simulink library "ControLibrary"  (R2015b)
settings: Solver=ode45  SolverMode=SingleTasking  StartTime=0.0  StopTime=10.0  RelTol=1e-3
values from neighbouring files (symbols this model uses):
  ControlSampleTime = 1/8000    (= 0.000125)    [initTPHardware.m]
  DCCC = initDCCC(LCL,SM)    [Sim_TP3_VSM_init.m]    (also in initDCCC.m = initHSS(LCL,SM))
undefined symbols (not defined in the file or in its folder): CCCTRL, DiscIntNeverNeededParam, VSMCTRL
undefined symbols (not defined in the file): HSS, VSMCC
libraries: FriedrichLibrary x46, simulink x23, simulink_extras x4, ControLibrary x2, ctrl_basic x2
(part 2 of 4)

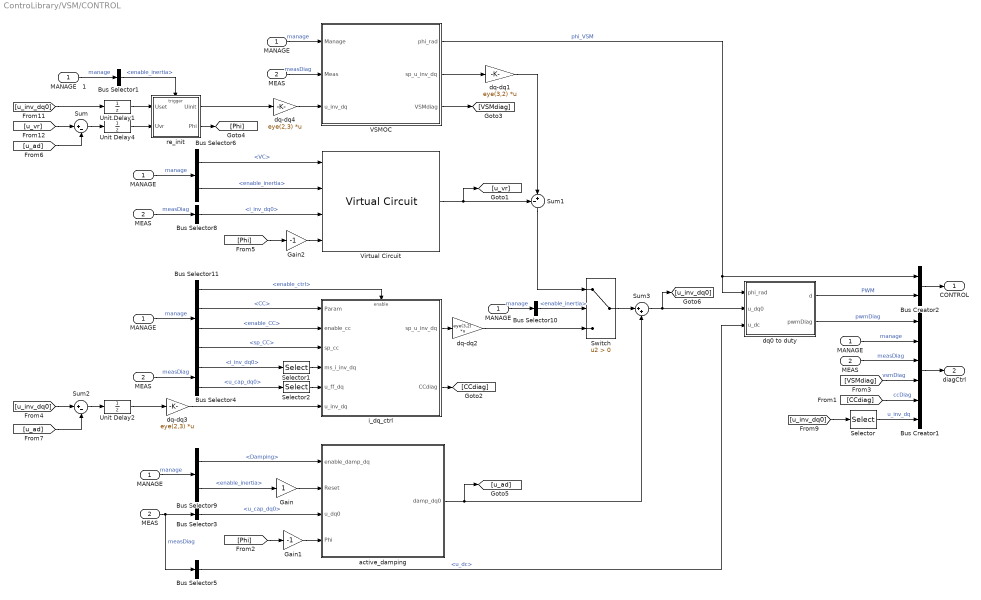
== system ControLibrary/VSM/CONTROL ==
  MANAGE : Inport
  MEAS : Inport  Port=2
  "  MANAGE " : InportShadow
  "  MEAS " : InportShadow  Port=2
  "  MEAS  " : InportShadow  Port=2
  " MANAGE" : InportShadow
  " MEAS" : InportShadow  Port=2
  Bus Creator1 : BusCreator  Inputs=6
  Bus Creator2 : BusCreator  Inputs=2
  Bus Selector1 : BusSelector  OutputSignals=enable_VSM.enable_inertia
  Bus Selector10 : BusSelector  OutputSignals=enable_VSM.enable_inertia
  Bus Selector11 : BusSelector  OutputSignals=enable_VSM.enable_ctrl,Param.CC,enable_CC,sp_CC
  Bus Selector3 : BusSelector  OutputSignals=u_cap.u_cap_dq0
  Bus Selector4 : BusSelector  OutputSignals=i_inv.i_inv_dq0,u_cap.u_cap_dq0
  Bus Selector5 : BusSelector  OutputSignals=u_dc
  Bus Selector6 : BusSelector  OutputSignals=Param.VC,enable_VSM.enable_inertia
  Bus Selector8 : BusSelector  OutputSignals=i_inv.i_inv_dq0
  Bus Selector9 : BusSelector  OutputSignals=Param.Damping,enable_VSM.enable_inertia
  Gain : Gain
  Gain1 : Gain  Gain=-1
  Gain2 : Gain  Gain=-1
  "MANAGE  " : InportShadow
  "MANAGE   " : InportShadow
  "MANAGE    " : InportShadow
  MANAGE   1 : InportShadow
  "MEAS " : InportShadow  Port=2
  Selector : Selector  InputPortWidth=3  IndexOptions=Index vector (dialog)  Indices=[1 2]  OutputSizes=1
  Selector1 : Selector  InputPortWidth=3  IndexOptions=Index vector (dialog)  Indices=[1 2]  OutputSizes=1
  Selector2 : Selector  InputPortWidth=3  IndexOptions=Index vector (dialog)  Indices=[1 2]  OutputSizes=1
  Sum : Sum  Inputs=|+-
  Sum1 : Sum  Inputs=-+|
  Sum2 : Sum  Inputs=|+-
  Sum3 : Sum  Inputs=|++
  Switch : Switch  Criteria=u2 > Threshold
  Unit Delay1 : UnitDelay  SampleTime=ControlSampleTime
  Unit Delay2 : UnitDelay  SampleTime=ControlSampleTime
  Unit Delay4 : UnitDelay  SampleTime=ControlSampleTime
  VSMOC : Subsystem  mask(VSM mit OC){VSM=Ctrl.VSM}
      mask prompts: VSM "VSM Parameter"
      mask help:
      | VSM(.Ta, .kpf, .kdf, .f0, .ku, .Tu)
      |
      | Parameter nicht auf der Maske:
      | ControlSampleTime
  Virtual Circuit : ControLibrary/Virtual Circuit
  active_damping : Subsystem  mask(Lead Lag){OmLead=Ctrl.VTFF.OmLead, OmLag=Ctrl.VTFF.OmLag}
      mask prompts: OmLead "Omega Lead"; OmLag "Omega Lag"
  dq-dq1 : Gain  Gain=eye(3,2)  Multiplication=Matrix(K*u)
  dq-dq2 : Gain  Gain=eye(3,2)  Multiplication=Matrix(K*u)
  dq-dq3 : Gain  Gain=eye(2,3)  Multiplication=Matrix(K*u)
  dq-dq4 : Gain  Gain=eye(2,3)  Multiplication=Matrix(K*u)
  dq0 to duty : Subsystem
  i_dq_ctrl : Subsystem  mask(PI DQ Stromregler){Kp=Ctrl.CC.kp, Ki=Ctrl.CC.ki, L_inv=Ctrl.CC.xff, Kff=Ctrl.CC.Kff}
      mask prompts: Kp "P-Anteil:"; Ki "I-Anteil:"; L_inv "Induktivität [pu]:"; Kff "Vorsteuerung"
      mask help:
      | - in pu Einheiten
      | - 2-phasige DQ Regelung
      | - Entkopplung der d- und q-Achse
      | - Vorsteuerung der Kondensatorspannung
      | - Aktive Dämpfung der LC-Filter Resonanz
      | - Aktive Dämpfung der Zwischenkreis Spannung
  re_init : Subsystem
  CONTROL : Outport
  diagCtrl : Outport  Port=2
  wires:
  [u_ad] -> Sum2/2
  [u_inv_dq0] -> Sum2/1
  Sum2/1 -> Unit Delay2/1
  [u_ad] -> Sum/2
  Sum/1 -> Unit Delay4/1
  [u_vr] -> Sum/1
  [Phi] -> Gain2/1
  Gain2/1 -> Virtual Circuit/4
  Gain1/1 -> active_damping/4(Phi)
  Gain/1 -> active_damping/2(Reset)
  Bus Selector6/2 -> Virtual Circuit/2  "<enable_inertia>"
  Bus Selector9/2 -> Gain/1  "<enable_inertia>"
  Bus Selector3/1 -> active_damping/3(u_dq0)  "<u_cap_dq0>"
  active_damping/1(damp_dq0) -> Sum3/2, [u_ad]
  MANAGE   1/1 -> Bus Selector1/1  "manage"
  Unit Delay2/1 -> dq-dq3/1
  Virtual Circuit/1 -> [u_vr], Sum1/1
  Switch/1 -> Sum3/1
  VSMOC/1(phi_rad) -> dq0 to duty/1(phi_rad), Bus Creator2/1  "phi_VSM"
  Bus Selector6/1 -> Virtual Circuit/1  "<VC>"
  "MANAGE   "/1 -> Bus Selector6/1  "manage"
  "  MEAS  "/1 -> Bus Selector8/1  "measDiag"
  Selector/1 -> Bus Creator1/6  "u_inv_dq"
  dq-dq4/1 -> VSMOC/3(u_inv_dq)
  VSMOC/2(sp_u_inv_dq) -> dq-dq1/1
  Selector1/1 -> i_dq_ctrl/4(ms_i_inv_dq)
  Bus Selector5/1 -> dq0 to duty/3(u_dc)  "<u_dc>"
  Bus Selector8/1 -> Virtual Circuit/3  "<i_inv_dq0>"
  [CCdiag] -> Bus Creator1/5  "ccDiag"
  i_dq_ctrl/1(sp_u_inv_dq) -> dq-dq2/1
  "MANAGE  "/1 -> Bus Selector10/1  "manage"
  Bus Selector10/1 -> Switch/2  "<enable_inertia>"
  i_dq_ctrl/2(CCdiag) -> [CCdiag]
  Bus Selector4/2 -> Selector2/1  "<u_cap_dq0>"
  Bus Selector4/1 -> Selector1/1  "<i_inv_dq0>"
  "MEAS "/1 -> Bus Selector4/1  "measDiag"
  "MANAGE    "/1 -> Bus Selector11/1  "manage"
  Bus Selector11/1 -> i_dq_ctrl/Enable  "<enable_ctrl>"
  Bus Selector11/3 -> i_dq_ctrl/2(enable_cc)  "<enable_CC>"
  Bus Selector11/4 -> i_dq_ctrl/3(sp_cc)  "<sp_CC>"
  Selector2/1 -> i_dq_ctrl/5(u_ff_dq)
  Bus Selector11/2 -> i_dq_ctrl/1(Param)  "<CC>"
  dq-dq3/1 -> i_dq_ctrl/6(u_inv_dq)
  [u_inv_dq0] -> Selector/1
  MEAS/1 -> VSMOC/2(Meas)  "measDiag"
  Bus Creator2/1 -> CONTROL/1
  " MEAS"/1 -> Bus Selector5/1, Bus Selector3/1  "measDiag"
  "  MANAGE "/1 -> Bus Creator1/2  "manage"
  Bus Creator1/1 -> diagCtrl/1
  Bus Selector9/1 -> active_damping/1(enable_damp_dq)  "<Damping>"
  " MANAGE"/1 -> Bus Selector9/1  "manage"
  dq0 to duty/2(pwmDiag) -> Bus Creator1/1  "pwmDiag"
  MANAGE/1 -> VSMOC/1(Manage)  "manage"
  dq0 to duty/1(d) -> Bus Creator2/2  "PWM"
  VSMOC/3(VSMdiag) -> [VSMdiag]
  "  MEAS "/1 -> Bus Creator1/3  "measDiag"
  [VSMdiag] -> Bus Creator1/4  "vsmDiag"
  Sum3/1 -> dq0 to duty/2(u_dq0), [u_inv_dq0]
  Sum1/1 -> Switch/1
  dq-dq1/1 -> Sum1/2
  dq-dq2/1 -> Switch/3
  Bus Selector1/1 -> re_init/Trigger  "<enable_inertia>"
  re_init/1(Uinit) -> dq-dq4/1
  Unit Delay1/1 -> re_init/1(Uset)
  Unit Delay4/1 -> re_init/2(Uvr)
  [Phi] -> Gain1/1
  [u_inv_dq0] -> Unit Delay1/1
  re_init/2(Phi) -> [Phi]

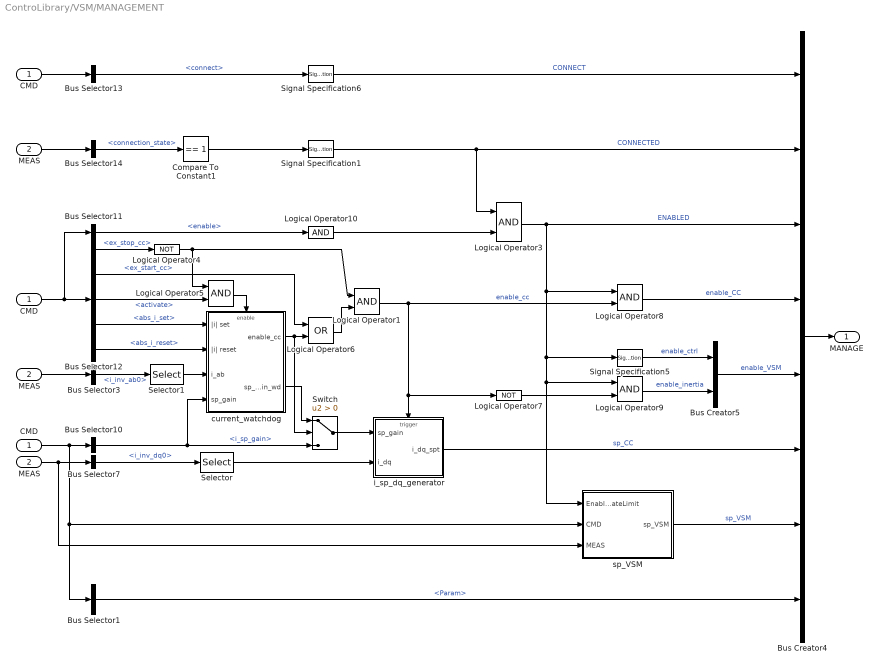
== system ControLibrary/VSM/MANAGEMENT ==
  CMD : Inport
  MEAS : Inport  Port=2
  "    MEAS   " : InportShadow  Port=2
  "  CMD  " : InportShadow
  " CMD" : InportShadow
  Bus Creator4 : BusCreator  Inputs=8
  Bus Creator5 : BusCreator  Inputs=2
  Bus Selector1 : BusSelector  OutputSignals=Param
  Bus Selector3 : BusSelector  OutputSignals=i_inv.i_inv_ab0
  Bus Selector7 : BusSelector  OutputSignals=i_inv.i_inv_dq0
  Bus Selector10 : BusSelector  OutputSignals=Param.CC.i_sp_gain
  Bus Selector11 : BusSelector  OutputSignals=Manage.enable
  Bus Selector12 : BusSelector  OutputSignals=Param.CC.ex_stop_cc,Param.CC.ex_start_cc,Param.CC.watchdog.activate,Param.CC.watchdog.abs_i_set,Param.CC.watchdog.abs_i_reset
  Bus Selector13 : BusSelector  OutputSignals=Manage.connect
  Bus Selector14 : BusSelector  OutputSignals=connection_state
  Compare To Constant1 : simulink/Logic and Bit Operations/Compare To Constant  relop===  const=1  OutDataTypeStr=boolean
  Logical Operator{1,3,5,8..9} (5 alike) : Logic  AllPortsSameDT=off  OutDataTypeStr=boolean
  Logical Operator4 : Logic  Operator=NOT  AllPortsSameDT=off  OutDataTypeStr=boolean
  Logical Operator6 : Logic  Operator=OR  AllPortsSameDT=off  OutDataTypeStr=boolean
  Logical Operator7 : Logic  Operator=NOT  AllPortsSameDT=off  OutDataTypeStr=boolean
  Logical Operator10 : Logic  Inputs=1  AllPortsSameDT=off  OutDataTypeStr=boolean
  "MEAS " : InportShadow  Port=2
  Selector : Selector  InputPortWidth=3  IndexOptions=Index vector (dialog)  Indices=[1 2]  OutputSizes=1
  Selector1 : Selector  InputPortWidth=3  IndexOptions=Index vector (dialog)  Indices=[1 2]  OutputSizes=1
  Signal Specification1 : SignalSpecification
  Signal Specification5 : SignalSpecification
  Signal Specification6 : SignalSpecification
  Switch : Switch  Criteria=u2 > Threshold
  current_watchdog : Subsystem
  i_sp_dq_generator : Subsystem
  sp_VSM : Subsystem
  MANAGE : Outport
  wires:
  Bus Selector1/1 -> Bus Creator4/8  "<Param>"
  Switch/1 -> i_sp_dq_generator/1(sp_gain)
  current_watchdog/2(sp_gain_wd) -> Switch/1
  sp_VSM/1(sp_VSM) -> Bus Creator4/7  "sp_VSM"
  "    MEAS   "/1 -> Bus Selector7/1, sp_VSM/3(MEAS)
  Bus Selector10/1 -> Switch/3, current_watchdog/4(sp_gain)  "<i_sp_gain>"
  Bus Selector11/1 -> Logical Operator10/1  "<enable>"
  Bus Selector12/3 -> Logical Operator5/2  "<activate>"
  Logical Operator5/1 -> current_watchdog/Enable
  Bus Selector12/1 -> Logical Operator4/1  "<ex_stop_cc>"
  Bus Selector12/2 -> Logical Operator6/1  "<ex_start_cc>"
  Bus Selector12/4 -> current_watchdog/1(|i| set)  "<abs_i_set>"
  Bus Selector12/5 -> current_watchdog/2(|i| reset)  "<abs_i_reset>"
  "  CMD  "/1 -> Bus Selector10/1, sp_VSM/2(CMD), Bus Selector1/1
  Signal Specification1/1 -> Logical Operator3/1, Bus Creator4/2  "CONNECTED"
  Logical Operator10/1 -> Logical Operator3/2
  Signal Specification6/1 -> Bus Creator4/1  "CONNECT"
  Bus Selector13/1 -> Signal Specification6/1  "<connect>"
  CMD/1 -> Bus Selector13/1
  Compare To Constant1/1 -> Signal Specification1/1
  Logical Operator3/1 -> Logical Operator9/1, sp_VSM/1(EnableRateLimit), Signal Specification5/1, Logical Operator8/1, Bus Creator4/3  "ENABLED"
  MEAS/1 -> Bus Selector14/1
  Bus Selector14/1 -> Compare To Constant1/1  "<connection_state>"
  " CMD"/1 -> Bus Selector12/1, Bus Selector11/1
  Bus Selector7/1 -> Selector/1  "<i_inv_dq0>"
  current_watchdog/1(enable_cc) -> Logical Operator6/2, Switch/2
  Bus Selector3/1 -> Selector1/1  "<i_inv_ab0>"
  Logical Operator6/1 -> Logical Operator1/2
  "MEAS "/1 -> Bus Selector3/1
  Bus Creator4/1 -> MANAGE/1
  Logical Operator8/1 -> Bus Creator4/4  "enable_CC"
  Bus Creator5/1 -> Bus Creator4/5  "enable_VSM"
  Signal Specification5/1 -> Bus Creator5/1  "enable_ctrl"
  Logical Operator9/1 -> Bus Creator5/2  "enable_inertia"
  Logical Operator7/1 -> Logical Operator9/2
  i_sp_dq_generator/1(i_dq_spt) -> Bus Creator4/6  "sp_CC"
  Logical Operator1/1 -> i_sp_dq_generator/Trigger, Logical Operator7/1, Logical Operator8/2  "enable_cc"
  Selector/1 -> i_sp_dq_generator/2(i_dq)
  Selector1/1 -> current_watchdog/3(i_ab)
  Logical Operator4/1 -> Logical Operator1/1, Logical Operator5/1

== system ControLibrary/VSM/Meas ==
  note: VSM Reference Frame
  note: Ucap reference frame
  MEASIN : Inport
  "CONTROL " : Inport  Port=2
  Bus Creator : BusCreator  Inputs=4
  Bus Creator4 : BusCreator  Inputs=10
  Bus Selector : BusSelector  OutputSignals=meas_i_inverter,meas_u_cap,meas_u_out,meas_i_out,meas_vol_dc
  Bus Selector1 : BusSelector  OutputSignals=connection_state,enabled
  Bus Selector2 : BusSelector  OutputSignals=phi_VSM
  Gain{,1..3} (4 alike) : Gain  Gain=eye(3,NrChannels)  Multiplication=Matrix(K*u)
  InstantPowerPhN : FriedrichLibrary/Transformations/InstantPowerPhN
  "InstantPowerPhN " : FriedrichLibrary/Transformations/InstantPowerPhN
  PowerPu : Gain  Gain=2/3
  "PowerPu " : Gain  Gain=2/3
  "SI -> pu" : Subsystem  mask{PU=PU}
      mask prompts: PU "PU System"
      mask DialogControl ParameterGroupVar Prompt: Per Unit
  Signal Specification : SignalSpecification  Dimensions=1
  Signal Specification1 : SignalSpecification  Dimensions=1
  Signal Specification2 : SignalSpecification  Dimensions=3
  Signal Specification3 : SignalSpecification  Dimensions=1
  Symmetrical PLL : FriedrichLibrary/Discrete Stuff/Symmetrical PLL  Kp_PLL=PLL.kp  Ki_PLL=PLL.ki  Kd_PLL=0  Ts=ControlSampleTime
  f2omega : Gain  Gain=2*pi
  meas_i_inv : Subsystem
  meas_i_out : Subsystem
  meas_u_cap : Subsystem
  meas_u_out : Subsystem
  MEAS : Outport
  wires:
  meas_i_out/1(i_out_x) -> Bus Creator4/6  "i_out"
  Gain1/1 -> Symmetrical PLL/1, InstantPowerPhN/1, "InstantPowerPhN "/1, meas_u_cap/1(abc)
  "PowerPu "/1 -> Bus Creator4/9  "PQ_out"
  "InstantPowerPhN "/1 -> "PowerPu "/1
  Bus Selector2/1 -> meas_u_cap/2(phi), meas_u_out/2(phi), meas_i_inv/2(phi)  "<phi_VSM>"
  Bus Selector1/2 -> Bus Creator4/2  "<enabled>"
  Bus Selector1/1 -> Bus Creator4/1  "<connection_state>"
  Bus Creator4/1 -> MEAS/1
  Signal Specification3/1 -> Bus Creator4/10  "u_dc"
  "SI -> pu"/1(MeasOut) -> Bus Selector/1
  f2omega/1 -> Bus Creator/4  "omega"
  Signal Specification2/1 -> Bus Creator/1  "vdq"
  Signal Specification1/1 -> Bus Creator/2  "phi"
  Signal Specification/1 -> Bus Creator/3, f2omega/1  "f"
  "CONTROL "/1 -> Bus Selector2/1
  MEASIN/1 -> "SI -> pu"/1(MeasIn), Bus Selector1/1
  Bus Selector/5 -> Signal Specification3/1  "<meas_vol_dc>"
  Bus Selector/1 -> Gain/1  "<meas_i_inverter>"
  Symmetrical PLL/2 -> meas_i_out/2(phi), Signal Specification1/1  "phi"
  Symmetrical PLL/3 -> Signal Specification/1  "f"
  Symmetrical PLL/1 -> Signal Specification2/1  "vdq"
  Gain/1 -> meas_i_inv/1(abc), InstantPowerPhN/2
  Bus Selector/2 -> Gain1/1  "<meas_u_cap>"
  InstantPowerPhN/1 -> PowerPu/1
  meas_i_inv/1(i_inv_x) -> Bus Creator4/3  "i_inv"
  meas_u_cap/1(u_cap_x) -> Bus Creator4/4  "u_cap"
  Gain2/1 -> "InstantPowerPhN "/2, meas_i_out/1(abc)
  Bus Selector/4 -> Gain2/1  "<meas_i_out>"
  Bus Creator/1 -> Bus Creator4/7  "PLL"
  Bus Selector/3 -> Gain3/1  "<meas_u_out>"
  meas_u_out/1(u_out_x) -> Bus Creator4/5  "u_out"
  Gain3/1 -> meas_u_out/1(abc)
  PowerPu/1 -> Bus Creator4/8  "PQ"

== system ControLibrary/VSMCC/BUS_GENERATION ==
  MANAGE : Inport
  CONTROL : Inport  Port=2
  Bus Creator1 : BusCreator  Inputs=4
  Bus Selector2 : BusSelector  OutputSignals=PWM
  Bus Selector3 : BusSelector  OutputSignals=ENABLED,CONNECT
  Bus Selector4 : BusSelector  OutputSignals=ENABLED,CONNECTED
  Bus Selector5 : BusSelector  OutputSignals=PWM
  Bus Creator6 : BusCreator  Inputs=4
  Data Type Conversion : DataTypeConversion
  Data Type Conversion1 : DataTypeConversion
  Ground : Ground
  Signal Specification{1..2,5..7} (5 alike) : SignalSpecification
  additional data1 : Constant  Value=0
  ctrl : Outport
  feedback : Outport  Port=2
  wires:
  Signal Specification6/1 -> Bus Creator6/2  "connected"
  Bus Selector3/2 -> Data Type Conversion1/1  "<CONNECT>"
  additional data1/1 -> Bus Creator1/4  "source_id"
  Data Type Conversion1/1 -> Bus Creator1/3  "connect"
  Data Type Conversion/1 -> Bus Creator1/2  "enable"
  Bus Selector3/1 -> Data Type Conversion/1  "<ENABLED>"
  Bus Creator6/1 -> feedback/1
  Bus Creator1/1 -> ctrl/1
  MANAGE/1 -> Bus Selector4/1, Bus Selector3/1
  Signal Specification7/1 -> Bus Creator6/3  "p_ack"
  Signal Specification1/1 -> Bus Creator1/1  "pwm"
  Signal Specification5/1 -> Bus Creator6/1  "enabled"
  CONTROL/1 -> Bus Selector5/1, Bus Selector2/1
  Bus Selector5/1 -> Signal Specification2/1  "<PWM>"
  Signal Specification2/1 -> Bus Creator6/4  "pwm"
  Bus Selector4/1 -> Signal Specification5/1  "<ENABLED>"
  Bus Selector4/2 -> Signal Specification6/1  "<CONNECTED>"
  Ground/1 -> Signal Specification7/1  "<P_ACK>"
  Bus Selector2/1 -> Signal Specification1/1  "<PWM>"

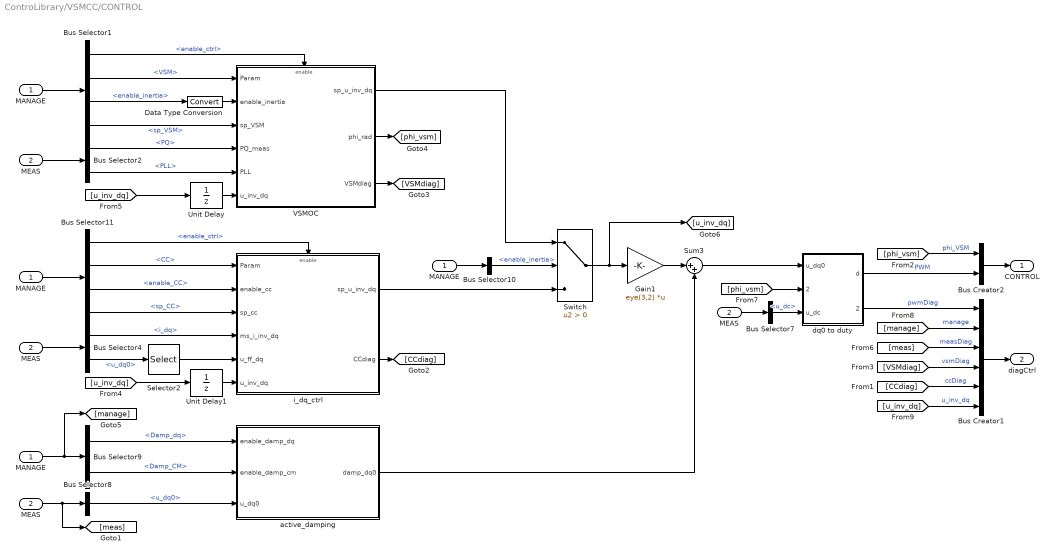
== system ControLibrary/VSMCC/CONTROL ==
  MANAGE : Inport
  MEAS : Inport  Port=2
  " MANAGE" : InportShadow
  " MEAS" : InportShadow  Port=2
  " MEAS  " : InportShadow  Port=2
  Bus Creator1 : BusCreator  Inputs=6
  Bus Creator2 : BusCreator  Inputs=2
  Bus Selector1 : BusSelector  OutputSignals=enable_VSM.enable_ctrl,Param.VSM,enable_VSM.enable_inertia,sp_VSM
  Bus Selector10 : BusSelector  OutputSignals=enable_VSM.enable_inertia
  Bus Selector11 : BusSelector  OutputSignals=enable_VSM.enable_ctrl,Param.CC,enable_CC,sp_CC
  Bus Selector2 : BusSelector  OutputSignals=PQ,PLL
  Bus Selector4 : BusSelector  OutputSignals=i_dq,u_dq0
  Bus Selector7 : BusSelector  OutputSignals=u_dc
  Bus Selector8 : BusSelector  OutputSignals=u_dq0
  Bus Selector9 : BusSelector  OutputSignals=Param.Damping.Damp_dq,Param.Damping.Damp_CM
  Data Type Conversion : DataTypeConversion
  Gain1 : Gain  Gain=eye(3,2)  Multiplication=Matrix(K*u)
  "MANAGE " : InportShadow
  "MANAGE  " : InportShadow
  "MEAS " : InportShadow  Port=2
  Selector2 : Selector  InputPortWidth=3  IndexOptions=Index vector (dialog)  Indices=[1 2]  OutputSizes=1
  Sum3 : Sum  Inputs=|++
  Switch : Switch  Criteria=u2 > Threshold
  Unit Delay : UnitDelay  InitialCondition=[1 0]  SampleTime=ControlSampleTime
  Unit Delay1 : UnitDelay  InitialCondition=[1 0]  SampleTime=ControlSampleTime
  VSMOC : Subsystem  mask(VSM mit OC){VSM=Ctrl.VSM}
      mask prompts: VSM "VSM Parameter"
      mask help:
      | VSM(.Ta, .kpf, .kdf, .f0, .ku, .Tu)
      |
      | Parameter nicht auf der Maske:
      | ControlSampleTime
  active_damping : Subsystem
  dq0 to duty : Subsystem
  i_dq_ctrl : Subsystem  mask(PI DQ Stromregler){Kp=Ctrl.CC.kp, Ki=Ctrl.CC.ki, L_inv=Ctrl.CC.xff, Kff=Ctrl.CC.Kff}
      mask prompts: Kp "P-Anteil:"; Ki "I-Anteil:"; L_inv "Induktivität [pu]:"; Kff "Vorsteuerung"
      mask help:
      | - in pu Einheiten
      | - 2-phasige DQ Regelung
      | - Entkopplung der d- und q-Achse
      | - Vorsteuerung der Kondensatorspannung
      | - Aktive Dämpfung der LC-Filter Resonanz
      | - Aktive Dämpfung der Zwischenkreis Spannung
  CONTROL : Outport
  diagCtrl : Outport  Port=2
  wires:
  VSMOC/1(sp_u_inv_dq) -> Switch/1
  VSMOC/2(phi_rad) -> [phi_vsm]
  Bus Selector7/1 -> dq0 to duty/3(u_dc)  "<u_dc>"
  " MEAS  "/1 -> Bus Selector7/1
  [meas] -> Bus Creator1/3  "measDiag"
  i_dq_ctrl/2(CCdiag) -> [CCdiag]
  Bus Selector4/2 -> Selector2/1  "<u_dq0>"
  MANAGE/1 -> Bus Selector1/1
  VSMOC/3(VSMdiag) -> [VSMdiag]
  MEAS/1 -> Bus Selector2/1
  Bus Selector4/1 -> i_dq_ctrl/4(ms_i_inv_dq)  "<i_dq>"
  dq0 to duty/1(d) -> Bus Creator2/2  "PWM"
  [VSMdiag] -> Bus Creator1/4  "vsmDiag"
  [CCdiag] -> Bus Creator1/5  "ccDiag"
  Bus Selector1/1 -> VSMOC/Enable  "<enable_ctrl>"
  dq0 to duty/2(pwmDiag) -> Bus Creator1/1  "pwmDiag"
  Bus Selector1/3 -> Data Type Conversion/1  "<enable_inertia>"
  "MEAS "/1 -> Bus Selector4/1
  "MANAGE "/1 -> Bus Selector11/1
  Bus Selector8/1 -> active_damping/3(u_dq0)  "<u_dq0>"
  " MANAGE"/1 -> [manage], Bus Selector9/1
  Bus Selector9/1 -> active_damping/1(enable_damp_dq)  "<Damp_dq>"
  Bus Selector9/2 -> active_damping/2(enable_damp_cm)  "<Damp_CM>"
  active_damping/1(damp_dq0) -> Sum3/2
  i_dq_ctrl/1(sp_u_inv_dq) -> Switch/3
  "MANAGE  "/1 -> Bus Selector10/1
  Bus Selector10/1 -> Switch/2  "<enable_inertia>"
  Sum3/1 -> dq0 to duty/1(u_dq0)
  [phi_vsm] -> dq0 to duty/2(phi_rad)
  Gain1/1 -> Sum3/1
  Bus Creator1/1 -> diagCtrl/1
  [manage] -> Bus Creator1/2  "manage"
  " MEAS"/1 -> [meas], Bus Selector8/1
  [phi_vsm] -> Bus Creator2/1  "phi_VSM"
  Bus Creator2/1 -> CONTROL/1
  Bus Selector1/2 -> VSMOC/1(Param)  "<VSM>"
  Data Type Conversion/1 -> VSMOC/2(enable_inertia)
  Bus Selector1/4 -> VSMOC/3(sp_VSM)  "<sp_VSM>"
  Bus Selector2/1 -> VSMOC/4(PQ_meas)  "<PQ>"
  Bus Selector2/2 -> VSMOC/5(PLL)  "<PLL>"
  [u_inv_dq] -> Unit Delay/1
  Bus Selector11/1 -> i_dq_ctrl/Enable  "<enable_ctrl>"
  Bus Selector11/3 -> i_dq_ctrl/2(enable_cc)  "<enable_CC>"
  Bus Selector11/4 -> i_dq_ctrl/3(sp_cc)  "<sp_CC>"
  Selector2/1 -> i_dq_ctrl/5(u_ff_dq)
  [u_inv_dq] -> Unit Delay1/1
  Switch/1 -> [u_inv_dq], Gain1/1
  Bus Selector11/2 -> i_dq_ctrl/1(Param)  "<CC>"
  [u_inv_dq] -> Bus Creator1/6  "u_inv_dq"
  Unit Delay/1 -> VSMOC/6(u_inv_dq)
  Unit Delay1/1 -> i_dq_ctrl/6(u_inv_dq)

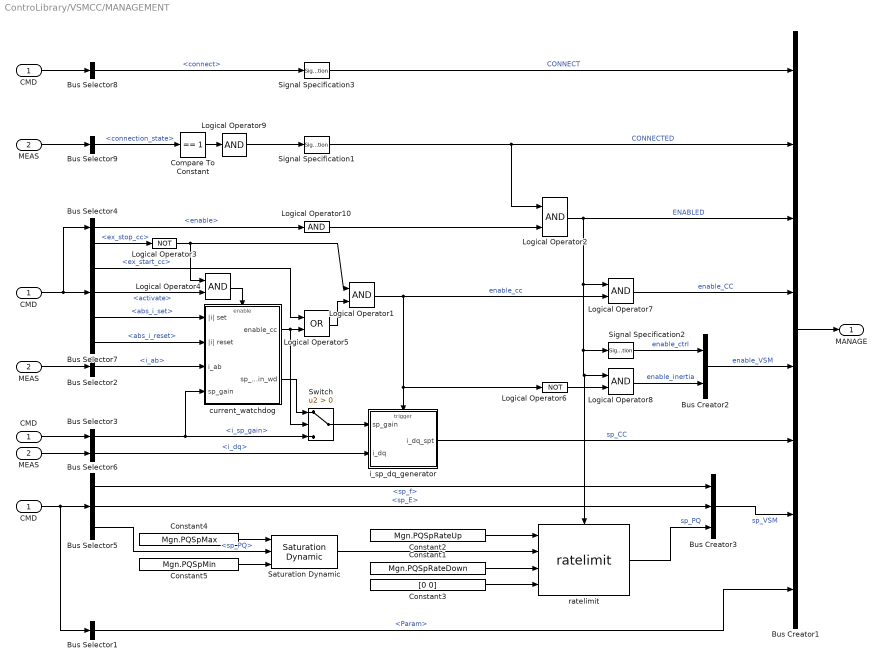
== system ControLibrary/VSMCC/MANAGEMENT ==
  CMD : Inport
  MEAS : Inport  Port=2
  "    MEAS   " : InportShadow  Port=2
  "  CMD  " : InportShadow
  " CMD" : InportShadow
  Bus Creator1 : BusCreator  Inputs=8
  Bus Creator2 : BusCreator  Inputs=2
  Bus Creator3 : BusCreator  Inputs=3
  Bus Selector1 : BusSelector  OutputSignals=Param
  Bus Selector2 : BusSelector  OutputSignals=i_ab
  Bus Selector5 : BusSelector  OutputSignals=Manage.VSM.sp_f,Manage.VSM.sp_E,Manage.VSM.sp_PQ
  Bus Selector6 : BusSelector  OutputSignals=i_dq
  Bus Selector3 : BusSelector  OutputSignals=Manage.CC.i_sp_gain
  Bus Selector4 : BusSelector  OutputSignals=Manage.Main.enable
  Bus Selector7 : BusSelector  OutputSignals=Manage.CC.ex_stop_cc,Manage.CC.ex_start_cc,Manage.CC.watchdog.activate,Manage.CC.watchdog.abs_i_set,Manage.CC.watchdog.abs_i_reset
  Bus Selector8 : BusSelector  OutputSignals=Manage.Main.connect
  Bus Selector9 : BusSelector  OutputSignals=connection_state
  "CMD " : InportShadow
  Compare To Constant : simulink/Logic and Bit Operations/Compare To Constant  relop===  const=1  OutDataTypeStr=boolean
  Constant1 : Constant  Value=Mgn.PQSpRateDown  SampleTime=ControlSampleTime
  Constant2 : Constant  Value=Mgn.PQSpRateUp  SampleTime=ControlSampleTime
  Constant3 : Constant  Value=[0 0]  SampleTime=ControlSampleTime
  Constant4 : Constant  Value=Mgn.PQSpMax  SampleTime=ControlSampleTime
  Constant5 : Constant  Value=Mgn.PQSpMin  SampleTime=ControlSampleTime
  Logical Operator{1..2,4,7..8} (5 alike) : Logic  AllPortsSameDT=off  OutDataTypeStr=boolean
  Logical Operator3 : Logic  Operator=NOT  AllPortsSameDT=off  OutDataTypeStr=boolean
  Logical Operator5 : Logic  Operator=OR  AllPortsSameDT=off  OutDataTypeStr=boolean
  Logical Operator6 : Logic  Operator=NOT  AllPortsSameDT=off  OutDataTypeStr=boolean
  Logical Operator10 : Logic  Inputs=1  AllPortsSameDT=off  OutDataTypeStr=boolean
  Logical Operator9 : Logic  Inputs=1  AllPortsSameDT=off  OutDataTypeStr=boolean
  "MEAS " : InportShadow  Port=2
  Saturation Dynamic : simulink/Discontinuities/Saturation Dynamic  OutMin=[]  OutMax=[]  OutDataTypeStr=Inherit: Same as second input  OutDataType=fixdt(1, 16)  OutScaling=2^-10  DoSatur=off
  Signal Specification1 : SignalSpecification
  Signal Specification2 : SignalSpecification
  Signal Specification3 : SignalSpecification
  Switch : Switch  Criteria=u2 > Threshold
  current_watchdog : Subsystem
  i_sp_dq_generator : Subsystem
  ratelimit : ControLibrary/ratelimit  Ts=ControlSampleTime
  MANAGE : Outport
  wires:
  "CMD "/1 -> Bus Selector1/1, Bus Selector5/1
  Bus Selector1/1 -> Bus Creator1/8  "<Param>"
  Logical Operator1/1 -> Logical Operator7/2, Logical Operator6/1, i_sp_dq_generator/Trigger  "enable_cc"
  i_sp_dq_generator/1(i_dq_spt) -> Bus Creator1/6  "sp_CC"
  Logical Operator6/1 -> Logical Operator8/2
  Logical Operator8/1 -> Bus Creator2/2  "enable_inertia"
  Signal Specification2/1 -> Bus Creator2/1  "enable_ctrl"
  Bus Creator2/1 -> Bus Creator1/5  "enable_VSM"
  Logical Operator7/1 -> Bus Creator1/4  "enable_CC"
  Bus Creator1/1 -> MANAGE/1
  "MEAS "/1 -> Bus Selector2/1
  Logical Operator5/1 -> Logical Operator1/2
  Bus Selector2/1 -> current_watchdog/3(i_ab)  "<i_ab>"
  current_watchdog/1(enable_cc) -> Switch/2, Logical Operator5/2
  Bus Selector6/1 -> i_sp_dq_generator/2(i_dq)  "<i_dq>"
  Logical Operator3/1 -> Logical Operator4/1, Logical Operator1/1
  " CMD"/1 -> Bus Selector4/1, Bus Selector7/1
  Bus Selector9/1 -> Compare To Constant/1  "<connection_state>"
  MEAS/1 -> Bus Selector9/1
  Logical Operator2/1 -> Bus Creator1/3, Signal Specification2/1, Logical Operator8/1, ratelimit/Enable, Logical Operator7/1  "ENABLED"
  Logical Operator9/1 -> Signal Specification1/1
  Compare To Constant/1 -> Logical Operator9/1
  CMD/1 -> Bus Selector8/1
  Bus Selector8/1 -> Signal Specification3/1  "<connect>"
  Signal Specification3/1 -> Bus Creator1/1  "CONNECT"
  Logical Operator10/1 -> Logical Operator2/2
  Signal Specification1/1 -> Logical Operator2/1, Bus Creator1/2  "CONNECTED"
  "  CMD  "/1 -> Bus Selector3/1
  Bus Selector7/5 -> current_watchdog/2(|i| reset)  "<abs_i_reset>"
  Bus Selector7/4 -> current_watchdog/1(|i| set)  "<abs_i_set>"
  Bus Selector7/2 -> Logical Operator5/1  "<ex_start_cc>"
  Bus Selector7/1 -> Logical Operator3/1  "<ex_stop_cc>"
  Logical Operator4/1 -> current_watchdog/Enable
  Bus Selector7/3 -> Logical Operator4/2  "<activate>"
  Bus Selector4/1 -> Logical Operator10/1  "<enable>"
  Bus Selector3/1 -> current_watchdog/4(sp_gain), Switch/3  "<i_sp_gain>"
  "    MEAS   "/1 -> Bus Selector6/1
  Constant2/1 -> ratelimit/1
  Constant1/1 -> ratelimit/3
  Bus Creator3/1 -> Bus Creator1/7  "sp_VSM"
  Constant3/1 -> ratelimit/4
  Bus Selector5/1 -> Bus Creator3/1  "<sp_f>"
  Bus Selector5/2 -> Bus Creator3/2  "<sp_E>"
  ratelimit/1 -> Bus Creator3/3  "sp_PQ"
  Saturation Dynamic/1 -> ratelimit/2
  Bus Selector5/3 -> Saturation Dynamic/2  "<sp_PQ>"
  Constant5/1 -> Saturation Dynamic/3
  Constant4/1 -> Saturation Dynamic/1
  current_watchdog/2(sp_gain_wd) -> Switch/1
  Switch/1 -> i_sp_dq_generator/1(sp_gain)

== system ControLibrary/VSMCC/Meas ==
  MEASIN : Inport
  "CONTROL " : Inport  Port=2
  Bus Creator : BusCreator  Inputs=4
  Bus Creator4 : BusCreator  Inputs=8
  Bus Selector : BusSelector  OutputSignals=meas_i_inverter,meas_u_cap,meas_vol_dc
  Bus Selector1 : BusSelector  OutputSignals=connection_state,enabled
  Bus Selector2 : BusSelector  OutputSignals=phi_VSM
  Gain : Gain  Gain=eye(3,NrChannels)  Multiplication=Matrix(K*u)
  Gain1 : Gain  Gain=eye(3,NrChannels)  Multiplication=Matrix(K*u)
  InstantPowerPhN : FriedrichLibrary/Transformations/InstantPowerPhN
  PhN->ab0 : FriedrichLibrary/Transformations/PhN->ab0  SystemSampleTime=-1
  PhN->ab2 : FriedrichLibrary/Transformations/PhN->ab0  SystemSampleTime=-1
  "SI -> pu" : Subsystem  mask{PU=PU}
      mask prompts: PU "PU System"
      mask DialogControl ParameterGroupVar Prompt: Per Unit
  Selector1 : Selector  InputPortWidth=3  IndexOptions=Index vector (dialog)  Indices=[1 2]  OutputSizes=1
  Selector2 : Selector  InputPortWidth=3  IndexOptions=Index vector (dialog)  Indices=[1 2]  OutputSizes=1
  Signal Specification : SignalSpecification  Dimensions=1
  Signal Specification1 : SignalSpecification  Dimensions=1
  Signal Specification2 : SignalSpecification  Dimensions=3
  Signal Specification3 : SignalSpecification  Dimensions=1
  Symmetrical PLL : FriedrichLibrary/Discrete Stuff/Symmetrical PLL  Kp_PLL=PLL.kp  Ki_PLL=PLL.ki  Kd_PLL=0  Ts=ControlSampleTime
  ab0->dq0-faster : FriedrichLibrary/Transformations/ab0->dq0-faster  SystemSampleTime=-1
  ab0->dq0-faster1 : FriedrichLibrary/Transformations/ab0->dq0-faster  SystemSampleTime=-1
  f-omega : Gain  Gain=2*pi
  MEAS : Outport
  wires:
  Selector2/1 -> Bus Creator4/4  "i_dq"
  ab0->dq0-faster1/1 -> Bus Creator4/5  "u_dq0"
  Bus Creator/1 -> Bus Creator4/6  "PLL"
  InstantPowerPhN/1 -> Bus Creator4/7  "PQ"
  Gain1/1 -> PhN->ab0/1, Symmetrical PLL/1, InstantPowerPhN/1
  Bus Selector/2 -> Gain1/1  "<meas_u_cap>"
  ab0->dq0-faster/1 -> Selector2/1
  PhN->ab2/1 -> Selector1/1, ab0->dq0-faster/1
  PhN->ab0/1 -> ab0->dq0-faster1/1
  Gain/1 -> PhN->ab2/1, InstantPowerPhN/2
  Symmetrical PLL/1 -> Signal Specification2/1  "vdq"
  Symmetrical PLL/3 -> Signal Specification/1  "f"
  Symmetrical PLL/2 -> Signal Specification1/1  "phi"
  Bus Selector/1 -> Gain/1  "<meas_i_inverter>"
  Bus Selector/3 -> Signal Specification3/1  "<meas_vol_dc>"
  MEASIN/1 -> Bus Selector1/1, "SI -> pu"/1(MeasIn)
  "CONTROL "/1 -> Bus Selector2/1
  Signal Specification/1 -> f-omega/1, Bus Creator/3  "f"
  Signal Specification1/1 -> Bus Creator/2  "phi"
  Signal Specification2/1 -> Bus Creator/1  "vdq"
  f-omega/1 -> Bus Creator/4  "omega"
  "SI -> pu"/1(MeasOut) -> Bus Selector/1
  Selector1/1 -> Bus Creator4/3  "i_ab"
  Signal Specification3/1 -> Bus Creator4/8  "u_dc"
  Bus Creator4/1 -> MEAS/1
  Bus Selector1/1 -> Bus Creator4/1  "<connection_state>"
  Bus Selector1/2 -> Bus Creator4/2  "<enabled>"
  Bus Selector2/1 -> ab0->dq0-faster1/2, ab0->dq0-faster/2  "<phi_VSM>"

== system ControLibrary/Virtual Circuit/Current Predictor ==
  u : Inport
  Delay : Delay  DelayLength=1  InitialCondition=0
  Sum : Sum  Inputs=|-+
  Sum1 : Sum  Inputs=|++
  y : Outport
  wires:
  Sum1/1 -> y/1
  Sum/1 -> Sum1/1
  Delay/1 -> Sum/1
  u/1 -> Delay/1, Sum1/2, Sum/2

== system ControLibrary/Virtual Circuit/PT1 ==
  U : Inport  SampleTime=Ts
  tau : Inport  Port=2  SampleTime=Ts
  Reset : Inport  Port=3  SampleTime=Ts
  Phi : Inport  Port=4
  Delay : Delay  DelayLength=1  InitialConditionSource=Input port  ExternalReset=Rising
      settings: InputPortMap=u0,r5,p4
  Divide : Product  Inputs=*/
  Gain : Gain  Gain=Ts
  Gain1 : Gain  Gain=K
  Saturation : Saturate  UpperLimit=inf  LowerLimit=Ts
  Sum : Sum  Inputs=|++
  Sum2 : Sum  Inputs=|+-
  Unit Delay2 : UnitDelay  InitialCondition=[0 0 0]  SampleTime=ControlSampleTime
  dq0->ab0 phi : FriedrichLibrary/Transformations/dq0->ab0 phi  SystemSampleTime=-1
  Y : Outport
  wires:
  dq0->ab0 phi/1 -> Delay/3
  Gain1/1 -> Y/1
  Sum2/1 -> Gain/1
  U/1 -> Sum2/1
  Gain/1 -> Divide/1
  Delay/1 -> Sum/2, Sum2/2
  tau/1 -> Saturation/1
  Divide/1 -> Sum/1
  Saturation/1 -> Divide/2
  Reset/1 -> Delay/2
  Sum/1 -> Delay/1, Unit Delay2/1, Gain1/1
  Unit Delay2/1 -> dq0->ab0 phi/1
  Phi/1 -> dq0->ab0 phi/2

== system ControLibrary/Virtual Circuit/PT2 ==
  U : Inport  SampleTime=Ts
  tau : Inport  Port=2  SampleTime=Ts
  Reset : Inport  Port=3  SampleTime=Ts
  Phi : Inport  Port=4
  Delay : Delay  DelayLength=1  InitialConditionSource=Input port  ExternalReset=Rising
      settings: InputPortMap=u0,r5,p4
  Divide : Product  Inputs=*/
  Gain : Gain  Gain=Ts
  Gain1 : Gain  Gain=K
  Saturation : Saturate  UpperLimit=inf  LowerLimit=Ts
  Sum : Sum  Inputs=|++
  Sum2 : Sum  Inputs=|+-
  Unit Delay2 : UnitDelay  InitialCondition=[0 0 0]  SampleTime=ControlSampleTime
  dq0->ab0 phi1 : FriedrichLibrary/Transformations/dq0->ab0 phi  SystemSampleTime=-1
  Y : Outport
  wires:
  Phi/1 -> dq0->ab0 phi1/2
  Unit Delay2/1 -> dq0->ab0 phi1/1
  Sum/1 -> Gain1/1, Unit Delay2/1, Delay/1
  Reset/1 -> Delay/2
  Saturation/1 -> Divide/2
  Divide/1 -> Sum/1
  tau/1 -> Saturation/1
  Delay/1 -> Sum2/2, Sum/2
  Gain/1 -> Divide/1
  U/1 -> Sum2/1
  Sum2/1 -> Gain/1
  Gain1/1 -> Y/1
  dq0->ab0 phi1/1 -> Delay/3

== system ControLibrary/cmd_CC/Damping ==
  Bus Creator1 : BusCreator  Inputs=4
  Tai1 : Constant  Value=CCCTRL.VTFF.EnableCM
  Tai2 : Constant  Value=CCCTRL.VTFF.EnableDQ
  Tai3 : Constant  Value=CCCTRL.VTFF.OmLag
  Tai4 : Constant  Value=CCCTRL.VTFF.OmLead
  Damping : Outport
  wires:
  Tai3/1 -> Bus Creator1/4  "OmLag"
  Tai4/1 -> Bus Creator1/3  "OmLead"
  Tai1/1 -> Bus Creator1/2  "Damp_CM"
  Bus Creator1/1 -> Damping/1
  Tai2/1 -> Bus Creator1/1  "Damp_dq"

== system ControLibrary/cmd_DCCC/CC Parameter ==
  Bus Creator1 : BusCreator  Inputs=5
  Kff : Constant  Value=DCCC.CC.Kff
  Tcc : Constant  Value=DCCC.CC.Tcc
  ki : Constant  Value=DCCC.CC.ki
  kp : Constant  Value=DCCC.CC.kp
  xff : Constant  Value=DCCC.CC.xff
  CC : Outport
  wires:
  Bus Creator1/1 -> CC/1
  Kff/1 -> Bus Creator1/1  "Kff"
  kp/1 -> Bus Creator1/3  "kp"
  ki/1 -> Bus Creator1/4  "ki"
  Tcc/1 -> Bus Creator1/2  "Tcc"
  xff/1 -> Bus Creator1/5  "xff"

== system ControLibrary/cmd_DCCC/Damping ==
  Bus Creator1 : BusCreator  Inputs=4
  Tai1 : Constant  Value=DCCC.VTFF.EnableCM
  Tai2 : Constant  Value=DCCC.VTFF.EnableDQ
  Tai3 : Constant  Value=DCCC.VTFF.OmLag
  Tai4 : Constant  Value=DCCC.VTFF.OmLead
  Damping : Outport
  wires:
  Tai3/1 -> Bus Creator1/4  "OmLag"
  Tai4/1 -> Bus Creator1/3  "OmLead"
  Tai1/1 -> Bus Creator1/2  "Damp_CM"
  Bus Creator1/1 -> Damping/1
  Tai2/1 -> Bus Creator1/1  "Damp_dq"

== system ControLibrary/cmd_DCCC/Manage ==
  Bus Creator : BusCreator  Inputs=3
  connect : Constant
  enable : Constant
  sp_DCbus_U : Constant  Value=720
  Manage : Outport
  wires:
  enable/1 -> Bus Creator/2  "enable"
  connect/1 -> Bus Creator/1  "connect"
  Bus Creator/1 -> Manage/1
  sp_DCbus_U/1 -> Bus Creator/3  "sp_DCbus_U"

== system ControLibrary/cmd_DCCC/VDC Parameter ==
  Bus Creator1 : BusCreator  Inputs=2
  ki : Constant  Value=DCCC.VDC.ki
  kp : Constant  Value=DCCC.VDC.kp
  VDC Param : Outport
  wires:
  ki/1 -> Bus Creator1/2  "ki"
  kp/1 -> Bus Creator1/1  "kp"
  Bus Creator1/1 -> VDC Param/1

== system ControLibrary/cmd_VSM template/Current Control ==
  note: else: init with u cap
  Bus Creator6 : BusCreator  Inputs=5
  Bus Creator7 : BusCreator  Inputs=3
  Init with u_inv [0/1] : Constant  Value=VSMCTRL.CC.init_uinv
  activate : Constant  Value=VSMCTRL.CC.activate
  external_stop_cc1 : Constant  Value=0
  external_stop_cc4 : Constant  Value=0
  i_reset_abs : Constant  Value=VSMCTRL.CC.i_reset
  i_set_abs : Constant  Value=VSMCTRL.CC.i_set
  i_sp_gain : Constant  Value=VSMCTRL.CC.i_sp_gain
  Current Control : Outport
  wires:
  Bus Creator6/1 -> Current Control/1  "CC"
  Init with u_inv [0/1]/1 -> Bus Creator6/1  "init_u_inv"
  external_stop_cc1/1 -> Bus Creator6/3  "ex_stop_cc"
  i_sp_gain/1 -> Bus Creator6/4  "i_sp_gain"
  i_set_abs/1 -> Bus Creator7/2  "abs_i_set"
  external_stop_cc4/1 -> Bus Creator6/2  "ex_start_cc"
  Bus Creator7/1 -> Bus Creator6/5  "watchdog"
  i_reset_abs/1 -> Bus Creator7/3  "abs_i_reset"
  activate/1 -> Bus Creator7/1  "activate"

== system ControLibrary/cmd_VSM template/Damping ==
  Bus Creator5 : BusCreator  Inputs=4
  EnableDamp_CM [0/1] : Constant  Value=VSMCTRL.VTFF.EnableCM
  EnableDamp_dq [0/1] : Constant  Value=VSMCTRL.VTFF.EnableDQ
  Omega Lag : Constant  Value=VSMCTRL.VTFF.OmLag
  Omega Lead : Constant  Value=VSMCTRL.VTFF.OmLead
  Damping : Outport
  wires:
  Omega Lag/1 -> Bus Creator5/4  "OmLag"
  Omega Lead/1 -> Bus Creator5/3  "OmLead"
  Bus Creator5/1 -> Damping/1
  EnableDamp_dq [0/1]/1 -> Bus Creator5/1  "Damp_dq"
  EnableDamp_CM [0/1]/1 -> Bus Creator5/2  "Damp_CM"

== system ControLibrary/cmd_VSM template/Manage ==
  Bus Creator : BusCreator  Inputs=2
  connect : Constant
  enable : Constant
  Manage : Outport
  wires:
  enable/1 -> Bus Creator/2  "enable"
  connect/1 -> Bus Creator/1  "connect"
  Bus Creator/1 -> Manage/1

== system ControLibrary/cmd_VSM template/Virtual Circuit ==
  Bus Creator9 : BusCreator  Inputs=7
  Virtual L1 : Constant  Value=VSMCTRL.VC.L1
  Virtual L1t : Constant  Value=VSMCTRL.VC.L1t
  Virtual R1 : Constant  Value=VSMCTRL.VC.R1
  Virtual R1t : Constant  Value=VSMCTRL.VC.R1t
  tau HP Slow : Constant  Value=VSMCTRL.VC.tauSlow
  tau Virtual L1 : Constant  Value=VSMCTRL.VC.tauL
  tau Virtual R1 : Constant  Value=VSMCTRL.VC.tauR
  Virtual Circuit : Outport
  wires:
  tau HP Slow/1 -> Bus Creator9/7  "tauS"
  tau Virtual L1/1 -> Bus Creator9/6  "tauL"
  tau Virtual R1/1 -> Bus Creator9/5  "tauR"
  Virtual L1/1 -> Bus Creator9/2  "L1"
  Bus Creator9/1 -> Virtual Circuit/1
  Virtual L1t/1 -> Bus Creator9/4  "L1t"
  Virtual R1t/1 -> Bus Creator9/3  "R1t"
  Virtual R1/1 -> Bus Creator9/1  "R1"

== system ControLibrary/cmd_VSM template/Virtual Synchronous Machine ==
  note: 0 Dekaktiviert Init Tiefpass
  note: 0 Dekaktiviert Init Tiefpass
  Bus Creator3 : BusCreator  Inputs=12
  E(sp_PQ) : Constant  Value=VSMCTRL.SP.E_comp
  Ta : Constant  Value=VSMCTRL.VSM.Ta
  Ta1 : Constant  Value=VSMCTRL.VSM.kpf
  Ta2 : Constant  Value=VSMCTRL.VSM.kdf
  Ta3 : Constant  Value=VSMCTRL.VSM.ku
  Ta4 : Constant  Value=VSMCTRL.VSM.Tu
  Ta5 : Constant  Value=0
  Ta6 : Constant  Value=0
  sp_E [pu] : Constant  Value=VSMCTRL.SP.E
  sp_PQ [pu] : Constant  Value=VSMCTRL.SP.PQ
  sp_PQ(U) limit : Constant  Value=VSMCTRL.SP.PQU_lim
  sp_f [Hz] : Constant  Value=VSMCTRL.SP.f
  Virtual Synchronous Machine : Outport
  wires:
  E(sp_PQ)/1 -> Bus Creator3/12  "sp_E_comp"
  Ta5/1 -> Bus Creator3/6  "Tuinit"
  Ta6/1 -> Bus Creator3/7  "TPinit"
  Ta1/1 -> Bus Creator3/2  "kpf"
  Ta2/1 -> Bus Creator3/3  "kdf"
  Ta3/1 -> Bus Creator3/4  "ku"
  Ta4/1 -> Bus Creator3/5  "Tu"
  Bus Creator3/1 -> Virtual Synchronous Machine/1
  Ta/1 -> Bus Creator3/1  "Ta"
  sp_PQ(U) limit/1 -> Bus Creator3/11  "sp_PQ_limit"
  sp_f [Hz]/1 -> Bus Creator3/8  "sp_f"
  sp_PQ [pu]/1 -> Bus Creator3/9  "sp_PQ"
  sp_E [pu]/1 -> Bus Creator3/10  "sp_E"

== system ControLibrary/CC/Grid Support/ PT1  ==
  u : Inport
  gain : Inport  Port=2
  T : Inport  Port=3
  Discrete-Time Integrator : DiscreteIntegrator  InitialConditionSource=external  InitialConditionSetting=State (most efficient)  SampleTime=ControlSampleTime  ICPrevOutput=DiscIntNeverNeededParam  ICPrevScaledInput=DiscIntNeverNeededParam
  Product1 : Product  Inputs=/*
  Product2 : Product  Inputs=**
  Sum : Sum  Inputs=|+-
  init : Constant  Value=0
  y : Outport
  wires:
  Sum/1 -> Product1/2
  Discrete-Time Integrator/1 -> Sum/2, y/1
  init/1 -> Discrete-Time Integrator/2
  u/1 -> Product2/1
  T/1 -> Product1/1
  Product1/1 -> Discrete-Time Integrator/1
  gain/1 -> Product2/2
  Product2/1 -> Sum/1

== system ControLibrary/CC/Grid Support/DT1 ==
  u : Inport
  gain : Inport  Port=2
  T : Inport  Port=3
  Discrete-Time Integrator : DiscreteIntegrator  InitialConditionSource=external  InitialConditionSetting=State (most efficient)  SampleTime=ControlSampleTime  ICPrevOutput=DiscIntNeverNeededParam  ICPrevScaledInput=DiscIntNeverNeededParam
  Divide1 : Product  Inputs=/*
  Product : Product
  Sum : Sum  Inputs=|+-
  Sum1 : Sum  Inputs=++|
  init1 : Constant  Value=0
  invert1 : Gain  Gain=-1
  y : Outport
  wires:
  gain/1 -> Product/2
  u/1 -> Product/1
  Product/1 -> invert1/1, Sum1/1
  Discrete-Time Integrator/1 -> Sum1/2
  init1/1 -> Sum/1
  invert1/1 -> Discrete-Time Integrator/2
  Sum/1 -> Discrete-Time Integrator/1
  Divide1/1 -> Sum/2, y/1
  T/1 -> Divide1/1
  Sum1/1 -> Divide1/2

== system ControLibrary/CC/Grid Support/PT1 tau_hf ==
  u : Inport
  Discrete-Time Integrator : DiscreteIntegrator  InitialConditionSource=external  InitialConditionSetting=State (most efficient)  SampleTime=ControlSampleTime  ICPrevOutput=DiscIntNeverNeededParam  ICPrevScaledInput=DiscIntNeverNeededParam
  Sum3 : Sum  Inputs=-+|
  Thochminus1 : Gain  Gain=1/T
  Thochminus2 : Gain  Gain=initU0
  y : Outport
  wires:
  u/1 -> Sum3/2, Thochminus2/1
  Sum3/1 -> Thochminus1/1
  Thochminus1/1 -> Discrete-Time Integrator/1
  Discrete-Time Integrator/1 -> y/1, Sum3/1
  Thochminus2/1 -> Discrete-Time Integrator/2

== system ControLibrary/CC/Grid Support/PT1  ==
  u : Inport
  gain : Inport  Port=2
  T : Inport  Port=3
  Discrete-Time Integrator : DiscreteIntegrator  InitialConditionSource=external  InitialConditionSetting=State (most efficient)  SampleTime=ControlSampleTime  ICPrevOutput=DiscIntNeverNeededParam  ICPrevScaledInput=DiscIntNeverNeededParam
  Product1 : Product  Inputs=/*
  Product2 : Product  Inputs=**
  Sum : Sum  Inputs=|+-
  init : Constant  Value=0
  y : Outport
  wires:
  Product2/1 -> Sum/1
  gain/1 -> Product2/2
  Product1/1 -> Discrete-Time Integrator/1
  T/1 -> Product1/1
  u/1 -> Product2/1
  init/1 -> Discrete-Time Integrator/2
  Discrete-Time Integrator/1 -> y/1, Sum/2
  Sum/1 -> Product1/2

== system ControLibrary/CC/Grid Support/PT1 tau_hf ==
  u : Inport
  Discrete-Time Integrator : DiscreteIntegrator  InitialConditionSource=external  InitialConditionSetting=State (most efficient)  SampleTime=ControlSampleTime  ICPrevOutput=DiscIntNeverNeededParam  ICPrevScaledInput=DiscIntNeverNeededParam
  Sum3 : Sum  Inputs=-+|
  Thochminus1 : Gain  Gain=1/T
  Thochminus2 : Gain  Gain=initU0
  y : Outport
  wires:
  Thochminus2/1 -> Discrete-Time Integrator/2
  Discrete-Time Integrator/1 -> Sum3/1, y/1
  Thochminus1/1 -> Discrete-Time Integrator/1
  Sum3/1 -> Thochminus1/1
  u/1 -> Thochminus2/1, Sum3/2

== system ControLibrary/DCCC/CONTROL/DCctrl ==
  Param : Inport
  w : Inport  Port=2
  x : Inport  Port=3
  umax : Inport  Port=4
  umin : Inport  Port=5
  x0 : Inport  Port=6
  Enable : EnablePort  StatesWhenEnabling=reset  ShowOutputPort=on
  Bus Creator2 : BusCreator  Inputs=3
  Bus Selector : BusSelector  OutputSignals=ki,kp
  Discrete-Time Integrator : DiscreteIntegrator  InitialConditionSource=external  InitialConditionSetting=State (most efficient)  SampleTime=ControlSampleTime  ICPrevOutput=DiscIntNeverNeededParam  ICPrevScaledInput=DiscIntNeverNeededParam
  Product : Product
  Product1 : Product
  Signal Specification : SignalSpecification  Dimensions=1
  Sum : Sum  Inputs=|+-
  Sum1 : Sum  Inputs=|+-
  Sum2 : Sum  Inputs=++|
  Sum3 : Sum  Inputs=+|+
  dynsat : simulink/Discontinuities/Saturation Dynamic  OutMin=[]  OutMax=[]  OutDataTypeStr=Inherit: Same as second input  OutDataType=fixdt(1, 16)  OutScaling=2^-10  DoSatur=off
  u : Outport
  ctrlDiag : Outport  Port=2
  wires:
  Param/1 -> Bus Selector/1
  Sum/1 -> Sum3/2, Product1/2
  Signal Specification/1 -> u/1
  Sum1/1 -> Sum3/1
  Sum3/1 -> Product/2
  Product/1 -> Discrete-Time Integrator/1
  w/1 -> [sp_u], Sum/1
  x/1 -> [ms_u], Sum/2
  Sum2/1 -> dynsat/2, Sum1/2
  dynsat/1 -> Sum1/1, Signal Specification/1
  umin/1 -> dynsat/3
  umax/1 -> dynsat/1
  x0/1 -> Discrete-Time Integrator/2
  Discrete-Time Integrator/1 -> Sum2/1
  Product1/1 -> Sum2/2
  [ms_u] -> Bus Creator2/3  "ms_u"
  [sp_u] -> Bus Creator2/2  "sp_u"
  Bus Creator2/1 -> ctrlDiag/1
  Enable/1 -> Bus Creator2/1  "enable"
  Bus Selector/1 -> Product/1  "<ki>"
  Bus Selector/2 -> Product1/1  "<kp>"

== system ControLibrary/DCCC/CONTROL/active_damping ==
  Param : Inport
  u_dq0 : Inport  Port=2
  Bus Selector : BusSelector  OutputSignals=Damp_dq,Damp_dq,Damp_CM,OmLead,OmLag
  Integrator (inertia) : DiscreteIntegrator  gainval=1  InitialCondition=1  InitialConditionSetting=State (most efficient)  SampleTime=ControlSampleTime  ICPrevOutput=DiscIntNeverNeededParam  ICPrevScaledInput=DiscIntNeverNeededParam
  Mux : Mux  Inputs=3
  Product{,1..3} (4 alike) : Product
  Sum : Sum  Inputs=|+-
  Sum2 : Sum  Inputs=++|
  damp_dq0 : Outport
  wires:
  Bus Selector/5 -> Product3/2  "<OmLag>"
  Bus Selector/4 -> Product2/1  "<OmLead>"
  Product2/1 -> Sum/1
  Integrator (inertia)/1 -> Sum2/2
  Product3/1 -> Sum/2
  Sum2/1 -> Product1/2, Product3/1
  Sum/1 -> Integrator (inertia)/1
  Param/1 -> Bus Selector/1
  Bus Selector/1 -> Mux/1  "<Damp_dq>"
  Bus Selector/2 -> Mux/2  "<Damp_dq>"
  Bus Selector/3 -> Mux/3  "<Damp_CM>"
  u_dq0/1 -> Product/2
  Product/1 -> Sum2/1, Product2/2
  Mux/1 -> Product/1, Product1/1  "enable"
  Product1/1 -> damp_dq0/1

== system ControLibrary/DCCC/CONTROL/dq0 to duty ==
  u_dq0 : Inport
  u_dc : Inport  Port=2
  phi_rad : Inport  Port=3
  Bias : Bias  Bias=Ctrl.PWM.tauT*PU.omegab
  Bus Creator3 : BusCreator  Inputs=1
  Divide : Product  Inputs=*/
  Gain : Gain  Gain=eye(NrChannels,3)  Multiplication=Matrix(K*u)
  Modulation : FriedrichLibrary/Transformations/Modulation  Method=Sine Modulation  Ts=ControlSampleTime
  Saturation : Saturate  UpperLimit=inf  LowerLimit=1
  Signal Specification1 : SignalSpecification
  dq0->ab0 phi : FriedrichLibrary/Transformations/dq0->ab0 phi  SystemSampleTime=-1
  d : Outport
  pwmDiag : Outport  Port=2
  wires:
  Bias/1 -> dq0->ab0 phi/2
  phi_rad/1 -> Bias/1
  u_dq0/1 -> dq0->ab0 phi/1
  Divide/1 -> Modulation/1  "ab0 norm"
  dq0->ab0 phi/1 -> Divide/1
  Modulation/1 -> Gain/1
  u_dc/1 -> Saturation/1
  Saturation/1 -> Divide/2
  Bus Creator3/1 -> pwmDiag/1  "pwmDiag"
  Gain/1 -> Bus Creator3/1, Signal Specification1/1  "pwm"
  Signal Specification1/1 -> d/1

== system ControLibrary/DCCC/CONTROL/i_dq_ctrl ==
  note: omega nicht berücksichtig
  Param : Inport
  sp_i_inv_dq : Inport  Port=2
  ms_i_inv_dq : Inport  Port=3
  ms_u_cap_dq : Inport  Port=4
  u_ff_dq : Inport  Port=5
  Enable : EnablePort  StatesWhenEnabling=reset
  Bus Creator2 : BusCreator  Inputs=5
  Bus Selector : BusSelector  OutputSignals=xff,kp,ki
  Discrete-Time Integrator : DiscreteIntegrator  InitialConditionSource=external  InitialConditionSetting=State (most efficient)  SampleTime=ControlSampleTime  ICPrevOutput=DiscIntNeverNeededParam  ICPrevScaledInput=DiscIntNeverNeededParam
  Gain3 : Gain  Gain=[0 -1 0;1 0 0;0 0 0]  Multiplication=Matrix(K*u)
  Product : Product
  Product1 : Product
  Product2 : Product
  Sum : Sum  Inputs=+++
  Sum1 : Sum  Inputs=-+-
  Sum3 : Sum  Inputs=-+|
  Sum5 : Sum
  sp_u_inv_dq : Outport
  ctrlDiag : Outport  Port=2
  wires:
  Bus Selector/1 -> Product2/2  "<xff>"
  Bus Selector/3 -> Product1/1  "<ki>"
  Bus Selector/2 -> Product/1  "<kp>"
  Param/1 -> Bus Selector/1
  Sum/1 -> sp_u_inv_dq/1
  Sum3/1 -> Product1/2, Product/2
  sp_i_inv_dq/1 -> [sp_i_dq], Sum3/2
  u_ff_dq/1 -> Sum1/3, [vff], Sum/3
  ms_u_cap_dq/1 -> Sum1/2
  [dqdcpl] -> Sum1/1
  Sum1/1 -> Discrete-Time Integrator/2
  Bus Creator2/1 -> ctrlDiag/1
  [sp_i_dq] -> Bus Creator2/1  "sp_i_dq"
  [i_dq] -> Bus Creator2/2  "i_dq"
  [piout] -> Bus Creator2/3  "piout"
  [vff] -> Bus Creator2/5  "vff"
  [dqdcpl] -> Bus Creator2/4  "dqdcpl"
  Gain3/1 -> [dqdcpl], Sum/1  "dq decouple"
  Sum5/1 -> Sum/2, [piout]  "pi ctrl"
  Discrete-Time Integrator/1 -> Sum5/2
  Product/1 -> Sum5/1
  Product1/1 -> Discrete-Time Integrator/1
  Product2/1 -> Gain3/1
  ms_i_inv_dq/1 -> Sum3/1, Product2/1, [i_dq]

== system ControLibrary/DCCC/MANAGEMENT/RateLimit ==
  sp_DCBus : Inport
  ms_dcbus : Inport  Port=2
  Enable : EnablePort  StatesWhenEnabling=reset
  Abs : Abs
  Abs1 : Abs
  Add : Sum  Inputs=+-
  Add1 : Sum  Inputs=+-
  Compare To Constant1 : simulink/Logic and Bit Operations/Compare To Constant  relop=<  const=1  OutDataTypeStr=boolean
  Compare To Constant2 : simulink/Logic and Bit Operations/Compare To Constant  relop=<  const=10  OutDataTypeStr=boolean
  Constant : Constant  Value=UDCbusSpRateUp  SampleTime=ControlSampleTime
  Constant1 : Constant  Value=UDCbusSpRateDown  SampleTime=ControlSampleTime
  Ground : Ground
  Logical Operator : Logic  AllPortsSameDT=off  OutDataTypeStr=boolean
  S-R Flip-Flop : simulink_extras/Flip Flops/S-R Flip-Flop  initial_condition=0
  Saturation Dynamic : simulink/Discontinuities/Saturation Dynamic  OutMin=[]  OutMax=[]  OutDataTypeStr=Inherit: Same as second input  OutDataType=fixdt(1, 16)  OutScaling=2^-10  DoSatur=off
  Terminator : Terminator
  Vdc max : Constant  Value=UDCbusSpMax  SampleTime=ControlSampleTime
  Vdc min : Constant  Value=UDCbusSpMin  SampleTime=ControlSampleTime
  ratelimit : Subsystem  mask{Ts=ControlSampleTime}
      mask DialogControl ParameterGroupVar Prompt: Rate Limiter
  sp_DCBus_slow : Outport
  DCBus_isset : Outport  Port=2
  wires:
  ms_dcbus/1 -> ratelimit/4(x0), Add1/2
  S-R Flip-Flop/1 -> DCBus_isset/1
  Ground/1 -> S-R Flip-Flop/2
  S-R Flip-Flop/2 -> Terminator/1
  Logical Operator/1 -> S-R Flip-Flop/1
  Compare To Constant2/1 -> Logical Operator/2
  Compare To Constant1/1 -> Logical Operator/1
  Abs1/1 -> Compare To Constant2/1
  Add1/1 -> Abs1/1
  Abs/1 -> Compare To Constant1/1
  Add/1 -> Abs/1
  Vdc max/1 -> Saturation Dynamic/1
  sp_DCBus/1 -> Saturation Dynamic/2
  Constant/1 -> ratelimit/1(rateup)
  Constant1/1 -> ratelimit/3(ratedown)
  Saturation Dynamic/1 -> ratelimit/2(x), Add/2
  ratelimit/1(x_slow) -> sp_DCBus_slow/1, Add/1, Add1/1
  Vdc min/1 -> Saturation Dynamic/3

== system ControLibrary/DCCC/Meas/SI -> pu ==
  MeasIn : Inport
  Bus Creator1 : BusCreator  Inputs=5
  Bus Selector : BusSelector  OutputSignals=meas_u_out,meas_i_out,meas_i_inverter,meas_u_dc,meas_u_cap
  Normalize : Gain  Gain=1/PU.Ub  OutDataTypeStr=double  RndMeth=Round
  Normalize1 : Gain  Gain=1/PU.Ib  OutDataTypeStr=double  RndMeth=Round
  Normalize2 : Gain  Gain=1/PU.Ib  OutDataTypeStr=double  RndMeth=Round
  Normalize3 : Gain  Gain=1/PU.Ub  OutDataTypeStr=double  RndMeth=Round
  Normalize4 : Gain  Gain=1/PU.Ub/2  OutDataTypeStr=double  RndMeth=Round
  MeasOut : Outport
  wires:
  Normalize3/1 -> Bus Creator1/5  "meas_u_cap"
  Bus Selector/5 -> Normalize3/1  "<meas_u_cap>"
  Bus Selector/4 -> Normalize4/1  "<meas_u_dc>"
  Bus Selector/3 -> Normalize1/1  "<meas_i_inverter>"
  Bus Selector/2 -> Normalize2/1  "<meas_i_out>"
  Bus Selector/1 -> Normalize/1  "<meas_u_out>"
  Bus Creator1/1 -> MeasOut/1
  Normalize4/1 -> Bus Creator1/4  "meas_vol_dc"
  Normalize2/1 -> Bus Creator1/2  "meas_i_out"
  Normalize1/1 -> Bus Creator1/3  "meas_i_inverter"
  Normalize/1 -> Bus Creator1/1  "meas_u_out"
  MeasIn/1 -> Bus Selector/1

== system ControLibrary/DCCC/Meas/meas_i_inv ==
  abc : Inport
  phi : Inport  Port=2
  PhN->ab2 : FriedrichLibrary/Transformations/PhN->ab0  SystemSampleTime=-1
  ab0->dq0-faster : FriedrichLibrary/Transformations/ab0->dq0-faster  SystemSampleTime=-1
  "abc " : Outport
  ab0 : Outport  Port=2
  dq0 : Outport  Port=3
  wires:
  ab0->dq0-faster/1 -> dq0/1  "i_dq"
  PhN->ab2/1 -> ab0->dq0-faster/1, ab0/1  "i_ab"
  abc/1 -> PhN->ab2/1, "abc "/1
  phi/1 -> ab0->dq0-faster/2

== system ControLibrary/DCCC/Meas/meas_i_out ==
  abc : Inport
  phi : Inport  Port=2
  PhN->ab2 : FriedrichLibrary/Transformations/PhN->ab0  SystemSampleTime=-1
  ab0->dq0-faster : FriedrichLibrary/Transformations/ab0->dq0-faster  SystemSampleTime=-1
  "abc " : Outport
  ab0 : Outport  Port=2
  dq0 : Outport  Port=3
  wires:
  phi/1 -> ab0->dq0-faster/2
  abc/1 -> "abc "/1, PhN->ab2/1
  PhN->ab2/1 -> ab0/1, ab0->dq0-faster/1  "i_ab"
  ab0->dq0-faster/1 -> dq0/1  "i_dq"

== system ControLibrary/DCCC/Meas/meas_u_cap ==
  abc : Inport
  phi : Inport  Port=2
  PhN->ab2 : FriedrichLibrary/Transformations/PhN->ab0  SystemSampleTime=-1
  ab0->dq0-faster : FriedrichLibrary/Transformations/ab0->dq0-faster  SystemSampleTime=-1
  "abc " : Outport
  ab0 : Outport  Port=2
  dq0 : Outport  Port=3
  wires:
  ab0->dq0-faster/1 -> dq0/1  "i_dq"
  PhN->ab2/1 -> ab0->dq0-faster/1, ab0/1  "i_ab"
  abc/1 -> PhN->ab2/1, "abc "/1
  phi/1 -> ab0->dq0-faster/2

== system ControLibrary/DCCC/Meas/meas_u_out ==
  abc : Inport
  phi : Inport  Port=2
  PhN->ab2 : FriedrichLibrary/Transformations/PhN->ab0  SystemSampleTime=-1
  ab0->dq0-faster : FriedrichLibrary/Transformations/ab0->dq0-faster  SystemSampleTime=-1
  "abc " : Outport
  ab0 : Outport  Port=2
  dq0 : Outport  Port=3
  wires:
  phi/1 -> ab0->dq0-faster/2
  abc/1 -> "abc "/1, PhN->ab2/1
  PhN->ab2/1 -> ab0/1, ab0->dq0-faster/1  "i_ab"
  ab0->dq0-faster/1 -> dq0/1  "i_dq"
